simulink model "TP3_ex_3"  (R2023a)
settings: Solver=ode1  StartTime=0.0  StopTime=2  FixedStep=0.001  RelTol=1e-3
undefined symbols (not defined in the file): DiscIntNeverNeededParam, K, ue, x0, xe
libraries: simulink x1
settings Model: Creator=abi7287  LastModifiedBy=abi7287

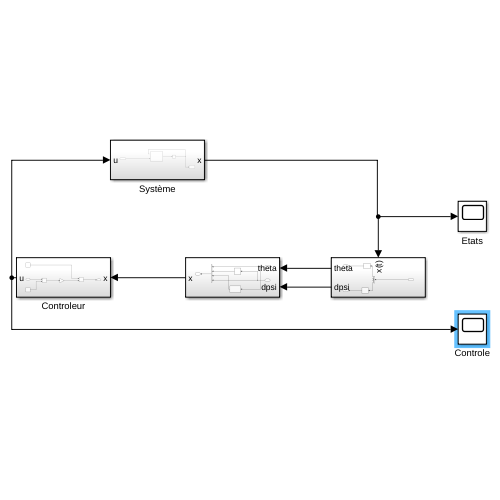
[thumbnail: Simulink's stored preview of the top-level diagram]
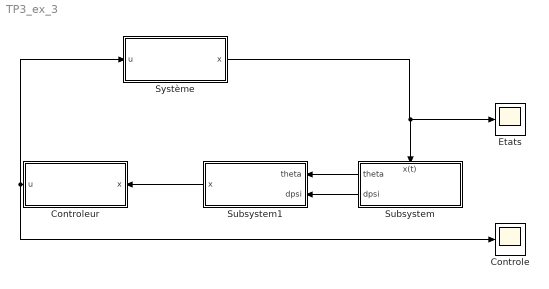
== system TP3_ex_3 ==
  Controle : Scope
  Controleur : Subsystem
  Etats : Scope
  Subsystem : Subsystem
      settings: PortSchema="{\"entries\":[{\"content\":{\"sides\":[{\"content\":{},\"type\":\"ConnectorPlacement.EquallySpacedRectSide\",\"uuid\":\"de52ba9e-0447-46ad-8d99-6c1b41871e5a\"},{\"content\":{\"connectorIds\":[\"Out1\",\"Out2\"],\"side\":\"RIGHT\"},\"type\":\"ConnectorPlacement.EquallySpacedRectSide\",\"uuid\":\"e34067f8-b8e8-46d9-9699-733de930604e\"},{\"content\":{\"connectorIds\":[\"In1\"],\"side\":\"TOP\"},\"type\":\"ConnectorPlacement.EquallySpacedRectSide\",\"uuid\":\"37c970e9-03d9-43a8-a452-c96cfb90c36f\"}]},\"type\":\"ConnectorPlacement.EquallySpacedConnector\",\"uuid\":\"f3e5dc2a-e39c-4eab-855e-72fd32e6738d\"}],\"packageUris\":[\"http://schema.mathworks.com/mf0/Connector/R2020b\"],\"version\":\"1.0\"}"
  Subsystem1 : Subsystem
  Système : Subsystem
  wires:
  Subsystem/2(dpsi) -> Subsystem1/2(dpsi)
  Subsystem/1(theta) -> Subsystem1/1(theta)
  Controleur/1(u) -> Controle/1, Système/1(u)
  Subsystem1/1(x) -> Controleur/1(x)
  Système/1(x) -> Subsystem/1(x(t)), Etats/1

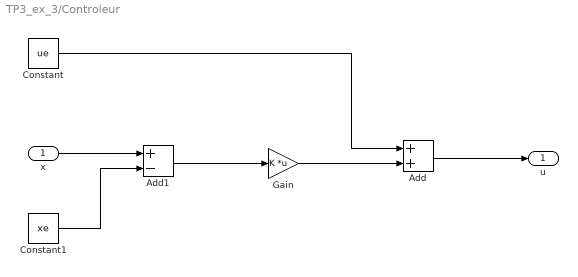
== system TP3_ex_3/Controleur ==
  x : Inport
  Add : Sum
  Add1 : Sum  Inputs=+-
  Constant : Constant  Value=ue
  Constant1 : Constant  Value=xe
  Gain : Gain  Gain=K  Multiplication=Matrix(K*u)
  u : Outport
  wires:
  Add/1 -> u/1
  Gain/1 -> Add/2
  Constant/1 -> Add/1
  Add1/1 -> Gain/1
  Constant1/1 -> Add1/2
  x/1 -> Add1/1

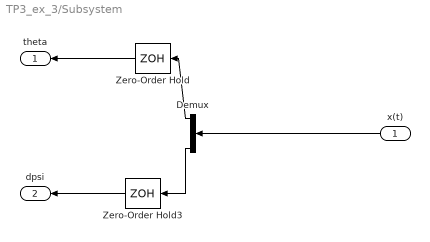
== system TP3_ex_3/Subsystem ==
  x(t) : Inport
  Demux : Demux
  Zero-Order Hold : ZeroOrderHold  SampleTime=-1
  Zero-Order Hold3 : ZeroOrderHold  SampleTime=-1
  theta : Outport
  dpsi : Outport  Port=2
  wires:
  Demux/1 -> Zero-Order Hold/1
  Demux/4 -> Zero-Order Hold3/1
  x(t)/1 -> Demux/1
  Zero-Order Hold/1 -> theta/1
  Zero-Order Hold3/1 -> dpsi/1

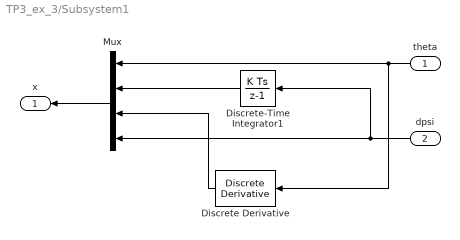
== system TP3_ex_3/Subsystem1 ==
  theta : Inport
  dpsi : Inport  Port=2
  Discrete Derivative : simulink/Discrete/Discrete Derivative  gainval=1.0  ICPrevScaledInput=0.0  OutMin=[]  OutMax=[]  OutDataType=fixdt(1, 16)  OutScaling=2^-10  DoSatur=off
  Discrete-Time Integrator1 : DiscreteIntegrator  InitialCondition=x0(2)  SampleTime=-1  ICPrevOutput=DiscIntNeverNeededParam  ICPrevScaledInput=DiscIntNeverNeededParam
  Mux : Mux
  x : Outport
  wires:
  theta/1 -> Discrete Derivative/1, Mux/1
  dpsi/1 -> Discrete-Time Integrator1/1, Mux/4
  Mux/1 -> x/1
  Discrete Derivative/1 -> Mux/3
  Discrete-Time Integrator1/1 -> Mux/2

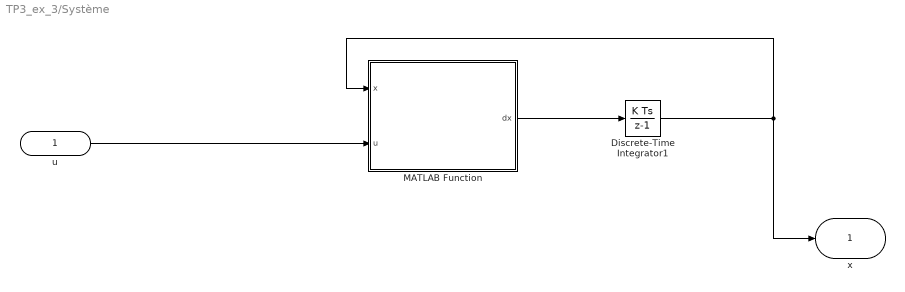
== system TP3_ex_3/Système ==
  u : Inport
  Discrete-Time Integrator1 : DiscreteIntegrator  InitialCondition=x0  SampleTime=-1  ICPrevOutput=DiscIntNeverNeededParam  ICPrevScaledInput=DiscIntNeverNeededParam
  MATLAB Function : MATLAB Function  TreatAsAtomicUnit=on
  x : Outport
  wires:
  u/1 -> MATLAB Function/2(u)
  Discrete-Time Integrator1/1 -> MATLAB Function/1(x), x/1
  MATLAB Function/1(dx) -> Discrete-Time Integrator1/1

== matlab function TP3_ex_3/Système/MATLAB Function ==
  data: x input; u input; dx output
function dx   = fonction( x, u)
%   Dynamic equations of motion of the segway on an axis.
%   Inputs: - x = [theta psi dtheta dpsi]
%               theta: average angle of the wheels      [rad]
%               psi: body pitch angle                   [rad]
%               dtheta: average velocity of the wheels  [rad/s]
%               dpsi: body pitch velocity               [rad/s]
%          - u: DC motor voltage (same value for both motors) [V]

    % State
    psi = x(2);
    dtheta = x(3);
    dpsi = x(4);

    % Parameters
    
    g = 9.81;           % gravity acceleration [m/sec^2]
    m = 0.03;           % wheel weight [kg]
    R = 0.04;           % wheel radius [m]
    Jw = m*R^2/2;       % wheel inertia moment [kg*m^2]
    M = 0.6;            % body weight [kg]
    H = 0.144;          % body height [m]
    L = H/2;            % distance of the center of mass from the wheel axle [m]
    Jpsi = M*L^2/3;     % body pitch inertia [kgm^2]
    Jm = 1e-5;          % DC motor inertia moment [kgm^2]
    Rm = 6.69;          % DC motor resistance [Ohm]
    Kb = 0.468;         % DC motor back EMF constant [Vsec/rad]
    Kt = 0.317;         % DC motor torque constant [Nm/A]
    n = 1;              % gear ratio
    fm = 0.0022;        % friction coefficient between body and DC motor
    fw = 0;             % friction coefficient between wheel and floor
    
    % Equations of motion
    c1 = (2*m+M)*R^2 + 2*Jw + 2*n^2*Jm;
    c2 = M*L*R*cos(psi) - 2*n^2*Jm;
    c3 = -M*L*R*dpsi^2*sin(psi);
    c4 = M*L^2 + Jpsi + 2*n^2*Jm;
    c5 = -M*g*L*sin(psi);

    alpha = Kt/Rm;
    beta = Kt*Kb/Rm + fm;

    Ftheta = alpha*(2*u) - 2*(beta+fw)*dtheta + 2*beta*dpsi;
    Fpsi = -alpha*(2*u) + 2*beta*dtheta - 2*beta*dpsi;

    ddtheta = (c4*c3 - c2*c5 + c4*Ftheta - c2*Fpsi)/(c4*c1 - c2^2);
    ddpsi = (Fpsi- c2*ddtheta - c5)/c4;
    dx = [dtheta dpsi ddtheta ddpsi]';

end
